simulink model "Maitri_RC"  (R2015a)
settings: Solver=ode45  StartTime=0.0  StopTime=inf  RelTol=1e-3
libraries: powerlib x8, simulink x1
settings Model: Creator=maitr  LastModifiedBy=maitr

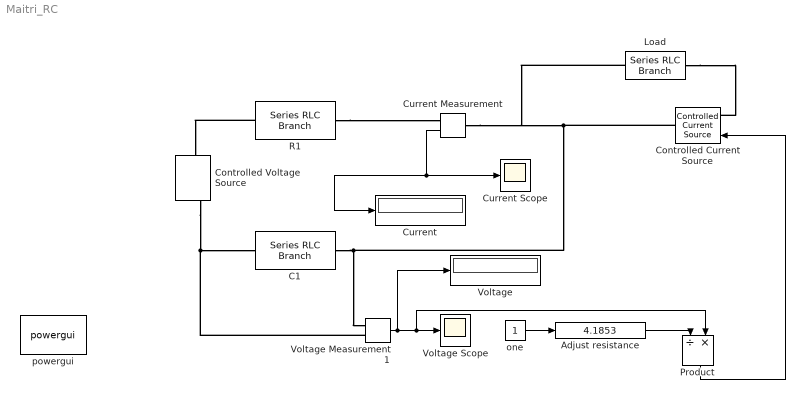
== system Maitri_RC ==
  Adjust resistance : simulink/Math Operations/Slider Gain  low=1  gain=4.1853  high=10.6
  C1 : powerlib/Elements/Series RLC Branch  LConnTagsString=__new0  RConnTagsString=__new0  BranchType=C  Resistance=1  Inductance=1e-3  SetiL0=off  InitialCurrent=0  Capacitance=10  Setx0=off  InitialVoltage=0  Measurements=None
  Controlled Current Source : powerlib/Electrical Sources/Controlled Current Source  Initialize=on  Source_Type=DC  Amplitude=0  Phase=0  Frequency=0  Measurements=None
  Controlled Voltage Source : powerlib/Electrical Sources/Controlled Voltage Source  Initialize=on  Source_Type=AC  Amplitude=400  Phase=0  Frequency=0  Measurements=None
  Current : Display
  Current Measurement : powerlib/Measurements/Current Measurement  PhasorSimulation=off  OutputType=Complex  PSBequivalent=0
  Current Scope : Scope
      settings: TimeRange=3600  YMin=0  YMax=10
  Load : powerlib/Elements/Series RLC Branch  LConnTagsString=__new0  RConnTagsString=__new0  BranchType=R  Resistance=1  Inductance=1e-3  SetiL0=off  InitialCurrent=0  Capacitance=1e-6  Setx0=off  InitialVoltage=0  Measurements=Branch voltage
  Product : Product  Inputs=/*  RndMeth=Zero
  R1 : powerlib/Elements/Series RLC Branch  LConnTagsString=__new0  RConnTagsString=__new0  BranchType=R  Resistance=550  Inductance=1e-3  SetiL0=off  InitialCurrent=0  Capacitance=1e-6  Setx0=off  InitialVoltage=0  Measurements=None
  Voltage : Display
  Voltage Measurement1 : powerlib/Measurements/Voltage Measurement  PhasorSimulation=off  OutputType=Complex  PSBequivalent=0
  Voltage Scope : Scope
      settings: TimeRange=3600  YMin=0  YMax=400
  one : Constant
  powergui : powerlib/powergui  Priority=1  SimulationMode=Discrete  SolverType=Tustin/Backward Euler (TBE)  SampleTime=0.0005  frequency=60  SPID=off  DisableSnubberDevices=off  DisableRonSwitches=off  DisableVfSwitches=off  SwTol=0  DisplayEquations=off  Interpol=off  methode=off  Ts=100  FunctionMessages=off  echomessages=off  HookPort=off  EnableUseOfTLC=off  x0status=blocks  frequencyindice=0  Pbase=100e6  ErrMax=1e-4  Iterations=50  UnitsV=kV  UnitsW=MW  buscounter=0  RestoreLinks=warning  ResistiveCurrentMeasurement=off  Frange=[0:2:500]  Ylog=off  Xlog=on  ShowGrid=off  save=off  variable=ZData  structure=0  ZoomFFT=off  StartTime=0.0  cycles=1  DisplayStyle=1  fundamental=60  FreqAxis=off  MaxFrequency=1000  frequencyindicesteady=1  RmsSteady=1  display=off
  wires:
  Adjust resistance/1 -> Product/1
  Product/1 -> Controlled Current Source/1
  one/1 -> Adjust resistance/1
  Voltage Measurement1/1 -> Voltage/1, Voltage Scope/1, Product/2
  Current Measurement/1 -> Current Scope/1, Current/1
  connections:
  R1/LConn1 -- Controlled Voltage Source/RConn1
  Controlled Voltage Source/LConn1 -- C1/LConn1 -- Voltage Measurement1/LConn2
  R1/RConn1 -- Current Measurement/RConn1
  C1/RConn1 -- Load/RConn1 -- Current Measurement/LConn1 -- Controlled Current Source/RConn1 -- Voltage Measurement1/LConn1
  Load/LConn1 -- Controlled Current Source/LConn1
